simulink model "sim1"  (R2022a)
settings: Solver=VariableStepAuto  StartTime=0.0  StopTime=10.0  RelTol=1e-3
settings Model: Creator=Mathias  LastModifiedBy=stump
settings DebuggingCC: UnconnectedInputMsg=warning  UnconnectedOutputMsg=warning  UnconnectedLineMsg=warning
settings RTWCC: DLArmComputeVersion=19.05

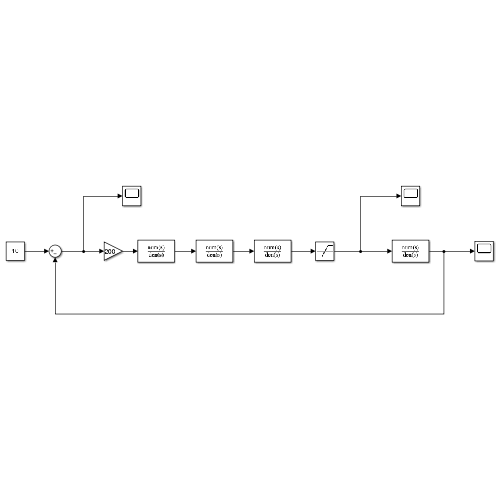
[thumbnail: Simulink's stored preview of the top-level diagram]
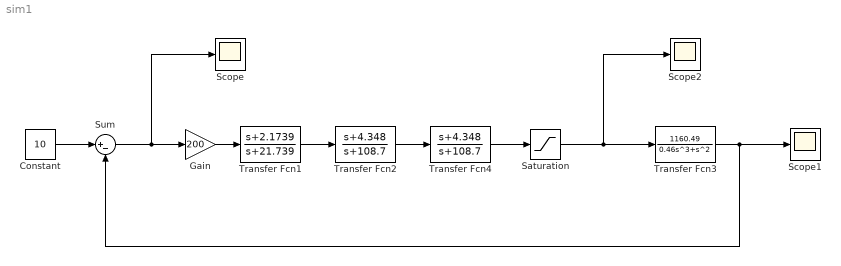
== system sim1 ==
  Constant : Constant  Value=10
  Gain : Gain  Gain=200
  Saturation : Saturate  UpperLimit=1  LowerLimit=-1
  Scope : Scope
  Scope1 : Scope
  Scope2 : Scope
  Sum : Sum  Inputs=|+-
  Transfer Fcn1 : TransferFcn  Numerator=[1,2.1739]  Denominator=[1,21.739]
  Transfer Fcn2 : TransferFcn  Numerator=[1,4.348]  Denominator=[1,108.7]
  Transfer Fcn3 : TransferFcn  Numerator=[1160.49]  Denominator=[0.46,1,0,0]
  Transfer Fcn4 : TransferFcn  Numerator=[1,4.348]  Denominator=[1,108.7]
  wires:
  Sum/1 -> Gain/1, Scope/1
  Transfer Fcn1/1 -> Transfer Fcn2/1
  Transfer Fcn2/1 -> Transfer Fcn4/1
  Transfer Fcn3/1 -> Scope1/1, Sum/2
  Gain/1 -> Transfer Fcn1/1
  Transfer Fcn4/1 -> Saturation/1
  Saturation/1 -> Scope2/1, Transfer Fcn3/1
  Constant/1 -> Sum/1
